simulink model "serial_i2c_severals_DS3231"  (R2016b)
settings: Solver=FixedStepDiscrete  StartTime=0.0  StopTime=10.0  FixedStep=1e-3  RelTol=1e-3
libraries: mbed_lib x4, mbed_i2c_several x1
settings Model: Creator=oh  LastModifiedBy=oh
settings DataIOCC: LimitDataPoints=on  SaveFormat=Array
settings OptimizationCC: LifeSpan=1
settings DebuggingCC: SFUnexpectedBacktrackingDiag=warning  SFNoUnconditionalDefaultTransitionDiag=warning  SFExecutionAtInitializationDiag=none
settings HardwareCC: ProdBitPerPointer=32  ProdBitPerSizeT=32  ProdBitPerPtrDiffT=32  ProdLargestAtomicInteger=Long  ProdLargestAtomicFloat=Double  ProdIntDivRoundTo=Undefined  ProdWordSize=32  ProdHWDeviceType=ARM Compatible->ARM Cortex
settings ModelReferenceCC: PropagateSignalLabelsOutOfModel=off
settings RTWCC: SystemTargetFile=mbed.tlc  TemplateMakefile=mbed.tmf  Description=Mbed Target (Embedded Target)  TargetLang=C++
settings CodeAppCC: IgnoreCustomStorageClasses=off
settings STFCustomTargetCC: TargetLibSuffix=.a  GenerateSampleERTMain=on  CombineOutputUpdateFcns=on  ERTCustomFileBanners=on  SupportContinuousTime=off  SupportNonInlinedSFcns=off  RemoveResetFunc=on  MATLABClassNameForMDSCustomization=Simulink.SoftwareTarget.ERTCustomization  GRTInterface=off  SystemTargetFile=mbed.tlc
settings ERTTargetCC: GenerateSampleERTMain=on  ParMdlRefBuildCompliant=off  CompOptLevelCompliant=off  ConcurrentExecutionCompliant=off  ERTFirstTimeCompliant=off  ModelStepFunctionPrototypeControlCompliant=off  CPPClassGenCompliant=off  UseToolchainInfoCompliant=off  ERTCustomFileTemplate=mbed_file_process.tlc  ConvertIfToSwitch=off  SuppressUnreachableDefaultCases=off
settings ConfigComp: CovMetricSettings=dw  CovHtmlReporting=on  CovSaveCumulativeToWorkspaceVar=on  CovSaveSingleToWorkspaceVar=on  CovExternalEMLEnable=off

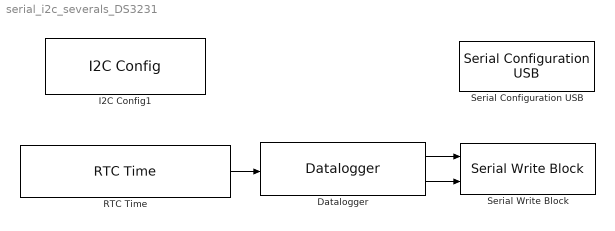
== system serial_i2c_severals_DS3231 ==
  Datalogger : mbed_lib/Utilities/Datalogger  TypeInputPorts={ 'uint32' 1 }  TypeOfInputs={'1*uint32'}  BufferSize=100  errEn=off  SampleTime=-1
  I2C Config1 : mbed_lib/Serial/I2C/I2C Config  Priority=0  I2CPort=1  Freq=100000  SDAPortName=B  SDAPinNumber=9  SCLPortName=B  SCLPinNumber=8
  RTC Time : mbed_i2c_several/RTC Time  i2cbus=1  SampleTime=1
  Serial Configuration USB : mbed_lib/Serial/UART/Serial Configuration USB  BaudRate=9600
  Serial Write Block : mbed_lib/Serial/UART/Serial Write Block  SerialPort=USB  numData=on  SampleTime=-1
  wires:
  RTC Time/1 -> Datalogger/1
  Datalogger/1 -> Serial Write Block/1
  Datalogger/2 -> Serial Write Block/2
